simulink model "pcm_tdm"  (R2023a)
settings: Solver=VariableStepAuto  StartTime=0.0  StopTime=1  RelTol=1e-3
libraries: simulink x4, dspquant2 x4, dspfdesign x2, dspsigops x2, dspindex x1
settings Model: Creator=dung  LastModifiedBy=dung

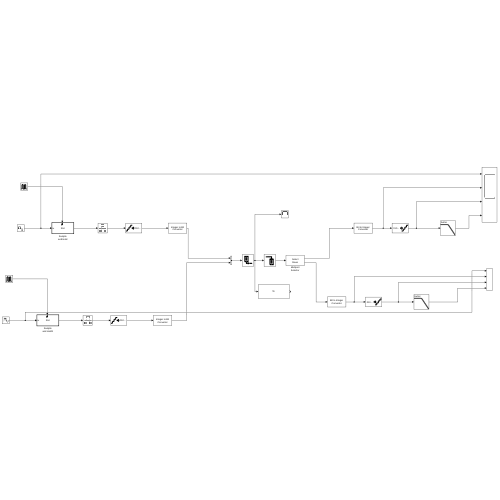
[thumbnail: Simulink's stored preview of the top-level diagram]
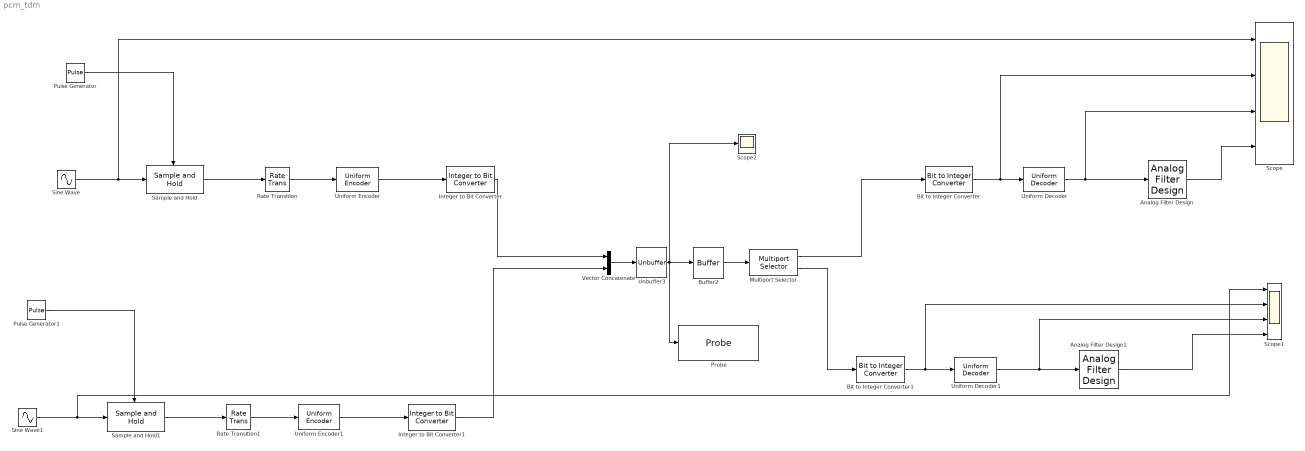
== system pcm_tdm ==
  Analog Filter Design : dspfdesign/Analog Filter Design  method=Butterworth  filttype=Lowpass  N=12  Wlo=2*pi*2100  Whi=80  Rp=2  Rs=40
  Analog Filter Design1 : dspfdesign/Analog Filter Design  method=Butterworth  filttype=Lowpass  N=12  Wlo=2*pi*1200  Whi=80  Rp=2  Rs=40
  Bit to Integer Converter : simulink/Logic and Bit Operations/Bit to Integer Converter  nbits=5  bitOrder=MSB first  signedOutputValues=Unsigned  outDtype=Inherit via internal rule  outDtypeSigned=Inherit via internal rule
  Bit to Integer Converter1 : simulink/Logic and Bit Operations/Bit to Integer Converter  nbits=5  bitOrder=MSB first  signedOutputValues=Unsigned  outDtype=Inherit via internal rule  outDtypeSigned=Inherit via internal rule
  Buffer2 : Buffer  N=10  OutputFrames=off
  Integer to Bit Converter : simulink/Logic and Bit Operations/Integer to Bit Converter  nbits=5  signedInputValues=Unsigned  bitOrder=MSB first  outDtype=Inherit via internal rule
  Integer to Bit Converter1 : simulink/Logic and Bit Operations/Integer to Bit Converter  nbits=5  signedInputValues=Unsigned  bitOrder=MSB first  outDtype=Inherit via internal rule
  Multiport Selector : dspindex/Multiport Selector  rowsOrCols=Rows  idxCellArray={ [1:5],[6:10]}  idxErrMode=Clip Index
      settings: LibrarySourceBlock=|
      | dsphdlsupportsigmgmt/Multiport
      | Selector
  Probe : Probe  ProbeWidth=off  ProbeComplexSignal=off
  Pulse Generator : DiscretePulseGenerator  PulseType=Time based  Period=1/8000  PulseWidth=50
  Pulse Generator1 : DiscretePulseGenerator  PulseType=Time based  Period=1/8000  PulseWidth=50
  Rate Transition : RateTransition  OutPortSampleTime=1/8000
  Rate Transition1 : RateTransition  OutPortSampleTime=1/8000
  Sample and Hold : dspsigops/Sample and Hold  trig=Rising edge  initCond=0  latchinput=off
  Sample and Hold1 : dspsigops/Sample and Hold  trig=Rising edge  initCond=0  latchinput=off
  Scope : Scope  NumInputPorts=4
  Scope1 : Scope  NumInputPorts=4
  Scope2 : Scope
  Sine Wave : Sin  Frequency=2*pi*2000  SampleTime=1/64000
  Sine Wave1 : Sin  Frequency=2*pi*1000  SampleTime=1/64000
  Unbuffer3 : Unbuffer  ic=10
  Uniform Decoder : dspquant2/Uniform Decoder  peak=1  bits=5  overflowMode=Saturate  otype=Double
  Uniform Decoder1 : dspquant2/Uniform Decoder  peak=1  bits=5  overflowMode=Saturate  otype=Double
  Uniform Encoder : dspquant2/Uniform Encoder  peak=1  bits=5  otype=Unsigned integer
  Uniform Encoder1 : dspquant2/Uniform Encoder  peak=1  bits=5  otype=Unsigned integer
  Vector Concatenate : Concatenate
  wires:
  Bit to Integer Converter/1 -> Scope/2, Uniform Decoder/1
  Analog Filter Design/1 -> Scope/4
  Uniform Decoder/1 -> Scope/3, Analog Filter Design/1
  Rate Transition/1 -> Uniform Encoder/1
  Sine Wave/1 -> Scope/1, Sample and Hold/1
  Uniform Encoder/1 -> Integer to Bit Converter/1
  Sample and Hold/1 -> Rate Transition/1
  Pulse Generator/1 -> Sample and Hold/Trigger
  Sine Wave1/1 -> Scope1/1, Sample and Hold1/1
  Rate Transition1/1 -> Uniform Encoder1/1
  Sample and Hold1/1 -> Rate Transition1/1
  Pulse Generator1/1 -> Sample and Hold1/Trigger
  Integer to Bit Converter1/1 -> Vector Concatenate/2
  Uniform Encoder1/1 -> Integer to Bit Converter1/1
  Bit to Integer Converter1/1 -> Scope1/2, Uniform Decoder1/1
  Uniform Decoder1/1 -> Scope1/3, Analog Filter Design1/1
  Integer to Bit Converter/1 -> Vector Concatenate/1
  Vector Concatenate/1 -> Unbuffer3/1
  Buffer2/1 -> Multiport Selector/1
  Analog Filter Design1/1 -> Scope1/4
  Multiport Selector/2 -> Bit to Integer Converter1/1
  Multiport Selector/1 -> Bit to Integer Converter/1
  Unbuffer3/1 -> Scope2/1, Probe/1, Buffer2/1
